simulink model "UniformQuantification"  (R2018b)
settings: Solver=VariableStepAuto  StartTime=0.0  StopTime=10.0  RelTol=1e-3
settings Model: Creator=Anderson  LastModifiedBy=Anderson

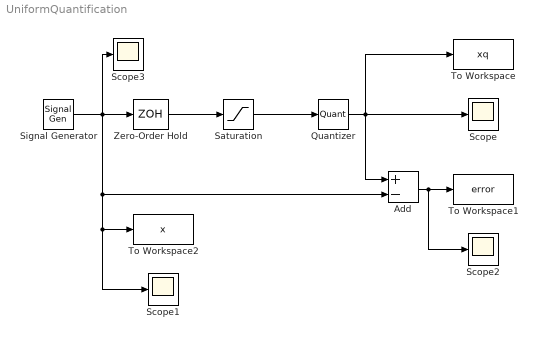
== system UniformQuantification ==
  Add : Sum  Inputs=+-
  Quantizer : Quantizer  QuantizationInterval=0.125
  Saturation : Saturate  UpperLimit=1  LowerLimit=-1
  Scope{,1..3} (4 alike) : Scope
  Signal Generator : SignalGenerator
  To Workspace : ToWorkspace  VariableName=xq  SaveFormat=Timeseries  SampleTime=-1
  To Workspace1 : ToWorkspace  VariableName=error  SaveFormat=Timeseries  SampleTime=-1
  To Workspace2 : ToWorkspace  VariableName=x  SaveFormat=Timeseries  SampleTime=-1
  Zero-Order Hold : ZeroOrderHold  SampleTime=0.01
  wires:
  Signal Generator/1 -> Scope3/1, To Workspace2/1, Scope1/1, Add/2, Zero-Order Hold/1
  Zero-Order Hold/1 -> Saturation/1
  Saturation/1 -> Quantizer/1
  Quantizer/1 -> To Workspace/1, Scope/1, Add/1
  Add/1 -> To Workspace1/1, Scope2/1
